simulink model "accelerometer"  (R2015a)
settings: Solver=ode45  StartTime=0.0  StopTime=10  RelTol=1e-3
model workspace (MAT data in the model file):
  randomSeed = 0
undefined symbols (not defined in the file): accelMax, accelOffset
libraries: simulink x1, dsparch4 x1
settings Model: ParameterArgumentNames=randomSeed  Creator=johnz  LastModifiedBy=johnz

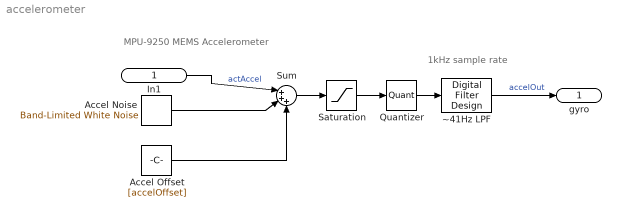
== system accelerometer ==
  note: MPU-9250 MEMS Accelerometer
  note: 1kHz sample rate
  In1 : Inport
  Accel Noise : simulink/Sources/Band-Limited White Noise  Cov=accelNoise  Ts=1/1000  seed=randomSeed
  Accel Offset : Constant  Value=[accelOffset]
  Quantizer : Quantizer  QuantizationInterval=accelSensitivity
  Saturation : Saturate  UpperLimit=accelMax  LowerLimit=-accelMax
  Sum : Sum  Inputs=|+++
  "~41Hz LPF " : dsparch4/Digital Filter Design  mwdsp_browser_bugfix_var=off
  gyro : Outport  OutDataTypeStr=double  PortDimensions=1
  wires:
  In1/1 -> Sum/1  "actAccel"
  Sum/1 -> Saturation/1
  Saturation/1 -> Quantizer/1
  Quantizer/1 -> "~41Hz LPF "/1
  Accel Offset/1 -> Sum/3
  "~41Hz LPF "/1 -> gyro/1  "accelOut"
  Accel Noise/1 -> Sum/2
